simulink model "example_3DOF_2"  (R2019a)
settings: Solver=ode45  StartTime=0.0  StopTime=250  RelTol=1e-5
PostLoadFcn:
  | flightControlCallback('initializeParameters', bdroot, '3DOF', 0);
InitFcn:
  | flightControlCallback('runSim', bdroot);
undefined symbols (not defined in the file or in its folder): aeroCoeff, vehicle
libraries: aerolibasang x3, shared3dof x1, sharedtransform x1
settings Model: Creator=Devansh  LastModifiedBy=Devansh
settings SolverCC: MinimalZcImpactIntegration=on
settings DataIOCC: ExternalInput=getinputstruct(op);  InitialState=getstatestruct(op);  SaveFormat=Array
settings OptimizationCC: EnhancedBackFolding=on  StrengthReduction=on  InitFltsAndDblsToZero=on  DifferentSizesBufferReuse=on
settings DebuggingCC: WriteAfterWriteMsg=DisableAll  AlgebraicLoopMsg=none  FcnCallInpInsideContextMsg=warning  UnconnectedInputMsg=none  UnconnectedOutputMsg=none  UnconnectedLineMsg=none  UniqueDataStoreMsg=error  StateNameClashWarn=warning  PregeneratedLibrarySubsystemCodeDiagnostic=none  StrictBusMsg=ErrorOnBusTreatedAsVector  SFUnexpectedBacktrackingDiag=warning  SFNoUnconditionalDefaultTransitionDiag=warning  SFExecutionAtInitializationDiag=none  ArithmeticOperatorsInVariantConditions=warning
settings ModelReferenceCC: PropagateSignalLabelsOutOfModel=off
settings SFSimCC: SimUseLocalCustomCode=off
settings RTWCC: RTWUseLocalCustomCode=off
settings CodeAppCC: StateflowObjectComments=on

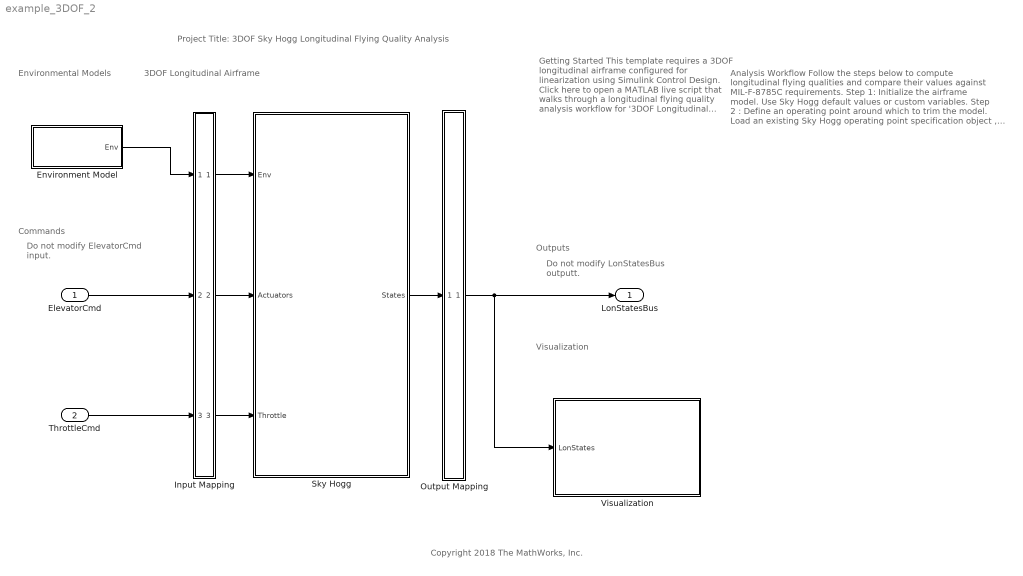
== system example_3DOF_2 ==
  note: Do not modify ElevatorCmd input.
  note: Project Title: 3DOF Sky Hogg Longitudinal Flying Quality Analysis
  note: Analysis Workflow
      | Follow the steps below to compute longitudinal flying qualities and compare their values against MIL-F-8785C requirements.
      |
      | Step 1: Initialize the airframe model. Use Sky Hogg default values or custom variables.
      |
      | Step 2 : Define an operating point around which to trim the model. Load an existing Sky Hogg operating point specification object , or launch the Linear Analysis Trim Tool to create a new one . You must use the 'Export' button in the dialog window to save your opCond.OperatingSpec object to the base workspace.
      |
      | Step 3: Trim the airframe model around a given operating point specification. (Optional:) Initialize the model with the trim inputs and states. Simulate the model to confirm steady-state behavior, then undo initialization.
      |
      | Step 4: Linearize the airframe dynamics around a trimmed operating point using the linear analysis input and output points defined in the model. You can modify linear analysis points by right-clicking on a signal line, and navigating to "Linear Analysis Points".
      |
      | Step 5: Compute longitudinal handling qualities (phugoid mode and short-period mode characteristics) for a linear airframe model using eigenvalue analysis, and compare the results against MIL-F-8785C requirements.
  note: Copyright 2018 The MathWorks, Inc.
  note: 3DOF Longitudinal Airframe
  note: Environmental Models
  note: Commands
  note: Visualization
  note: Outputs
  note: Getting Started
      | This template requires a 3DOF longitudinal airframe configured for linearization using Simulink Control Design.
      |
      | Click here to open a MATLAB live script that walks through a longitudinal flying quality analysis workflow for '3DOF Longitudinal Airframe' Simulink template .
  note: Do not modify LonStatesBus outputt.
  ElevatorCmd : Inport  OutDataTypeStr=double
  ThrottleCmd : Inport  Port=2  OutDataTypeStr=double
  Environment Model : Subsystem
  Input Mapping : Subsystem
  Output Mapping : Subsystem
  Sky Hogg : Subsystem
      settings: AttributesFormatString=|
      | Must contain one 3DOF
      | (Body Axis) block
  Visualization : Subsystem
  LonStatesBus : Outport
  wires:
  Sky Hogg/1(States) -> Output Mapping/1(StatesIn)
  Environment Model/1(Env) -> Input Mapping/1(EnvironmentIn)
  ElevatorCmd/1 -> Input Mapping/2(ActuatorCmds)
  ThrottleCmd/1 -> Input Mapping/3(ThrottleIn)
  Input Mapping/3(ThrottleOut) -> Sky Hogg/3(Throttle)
  Input Mapping/2(ActuatorCmdsOut) -> Sky Hogg/2(Actuators)
  Input Mapping/1(EnvironmentOut) -> Sky Hogg/1(Env)
  Output Mapping/1(StatesOut) -> Visualization/1(LonStates), LonStatesBus/1

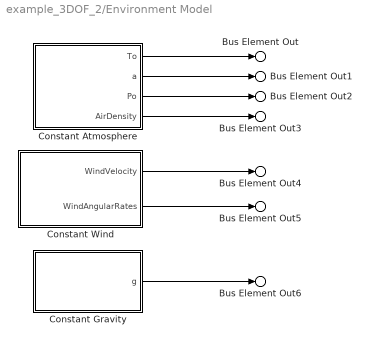
== system example_3DOF_2/Environment Model ==
  Constant Atmosphere : Subsystem  VariantControl=atmosCONST  mask(Standard Atmospheric Constants){To=275.15, a=332.529, Po=79495.2, AirDensity=1.00649}
      mask prompts: To "Constant Temperature (K):"; a "Constant Speed of Sound (m/s):"; Po "Constant Pressure (Pa):"; AirDensity "Constant Air Density (kg/m^3):"
  Constant Gravity : Subsystem  VariantControl=gravCONST  mask(Constant Gravitational Acceleration){g=[0 0 9.80665]}
      mask prompts: g "Constant Gravitational Acceleration (m/s^2):"
  Constant Wind : Subsystem  VariantControl=windCONST  mask(Constant Wind Values){ugvgwg=[-2 0 -1], pgqgrg=[0 0 0]}
      mask prompts: ugvgwg "Constant Wind Velocity (m/s):"; pgqgrg "Constant Wind Angular Rates (rad/s):"
  Bus Element Out : Outport  PortName=Env  Element=To
  Bus Element Out1 : Outport  PortName=Env  Element=a
  Bus Element Out2 : Outport  PortName=Env  Element=Po
  Bus Element Out3 : Outport  PortName=Env  Element=AirDensity
  Bus Element Out4 : Outport  PortName=Env  Element=WindVelocity
  Bus Element Out5 : Outport  PortName=Env  Element=WindAngularRates
  Bus Element Out6 : Outport  PortName=Env  Element=g
  wires:
  Constant Gravity/1(g) -> Bus Element Out6/1
  Constant Atmosphere/2(a) -> Bus Element Out1/1
  Constant Wind/1(WindVelocity) -> Bus Element Out4/1
  Constant Atmosphere/1(To) -> Bus Element Out/1
  Constant Atmosphere/4(AirDensity) -> Bus Element Out3/1
  Constant Atmosphere/3(Po) -> Bus Element Out2/1
  Constant Wind/2(WindAngularRates) -> Bus Element Out5/1

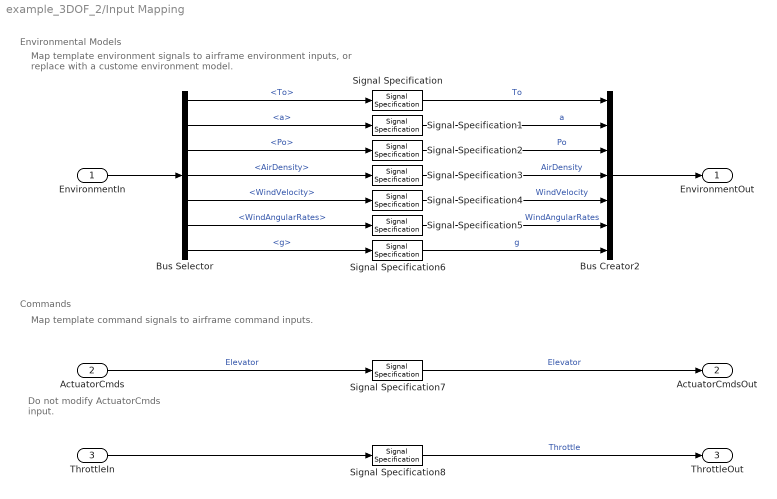
== system example_3DOF_2/Input Mapping ==
  note: Map template environment signals to airframe environment inputs, or replace with a custome environment model.
  note: Map template command signals to airframe command inputs.
  note: Commands
  note: Environmental Models
  note: Do not modify ActuatorCmds input.
  EnvironmentIn : Inport
  ActuatorCmds : Inport  Port=2
  ThrottleIn : Inport  Port=3
  Bus Creator2 : BusCreator  Inputs=7
  Bus Selector : BusSelector  OutputSignals=To,a,Po,AirDensity,WindVelocity,WindAngularRates,g
  Signal Specification{,1..8} (9 alike) : SignalSpecification  OutDataTypeStr=double
  EnvironmentOut : Outport
  ActuatorCmdsOut : Outport  Port=2
  ThrottleOut : Outport  Port=3
  wires:
  EnvironmentIn/1 -> Bus Selector/1
  Bus Creator2/1 -> EnvironmentOut/1
  ThrottleIn/1 -> Signal Specification8/1
  Bus Selector/1 -> Signal Specification/1  "<To>"
  Bus Selector/2 -> Signal Specification1/1  "<a>"
  Bus Selector/3 -> Signal Specification2/1  "<Po>"
  Bus Selector/4 -> Signal Specification3/1  "<AirDensity>"
  Bus Selector/5 -> Signal Specification4/1  "<WindVelocity>"
  Bus Selector/6 -> Signal Specification5/1  "<WindAngularRates>"
  Bus Selector/7 -> Signal Specification6/1  "<g>"
  ActuatorCmds/1 -> Signal Specification7/1  "Elevator"
  Signal Specification2/1 -> Bus Creator2/3  "Po"
  Signal Specification3/1 -> Bus Creator2/4  "AirDensity"
  Signal Specification6/1 -> Bus Creator2/7  "g"
  Signal Specification4/1 -> Bus Creator2/5  "WindVelocity"
  Signal Specification5/1 -> Bus Creator2/6  "WindAngularRates"
  Signal Specification/1 -> Bus Creator2/1  "To"
  Signal Specification1/1 -> Bus Creator2/2  "a"
  Signal Specification7/1 -> ActuatorCmdsOut/1  "Elevator"
  Signal Specification8/1 -> ThrottleOut/1  "Throttle"

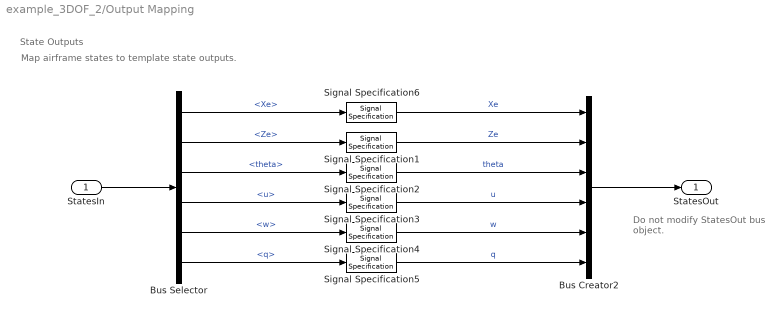
== system example_3DOF_2/Output Mapping ==
  note: State Outputs
  note: Map airframe states to template state outputs.
  note: Do not modify StatesOut bus object.
  StatesIn : Inport
  Bus Creator2 : BusCreator  Inputs=6
  Bus Selector : BusSelector  OutputSignals=Xe,Ze,theta,u,w,q
  Signal Specification{1..6} (6 alike) : SignalSpecification  OutDataTypeStr=double
  StatesOut : Outport  OutDataTypeStr=Bus: flightControl3DOFStatesBus
  wires:
  Bus Creator2/1 -> StatesOut/1
  StatesIn/1 -> Bus Selector/1
  Bus Selector/1 -> Signal Specification6/1  "<Xe>"
  Bus Selector/2 -> Signal Specification1/1  "<Ze>"
  Bus Selector/3 -> Signal Specification2/1  "<theta>"
  Bus Selector/4 -> Signal Specification3/1  "<u>"
  Bus Selector/5 -> Signal Specification4/1  "<w>"
  Bus Selector/6 -> Signal Specification5/1  "<q>"
  Signal Specification6/1 -> Bus Creator2/1  "Xe"
  Signal Specification1/1 -> Bus Creator2/2  "Ze"
  Signal Specification2/1 -> Bus Creator2/3  "theta"
  Signal Specification3/1 -> Bus Creator2/4  "u"
  Signal Specification4/1 -> Bus Creator2/5  "w"
  Signal Specification5/1 -> Bus Creator2/6  "q"

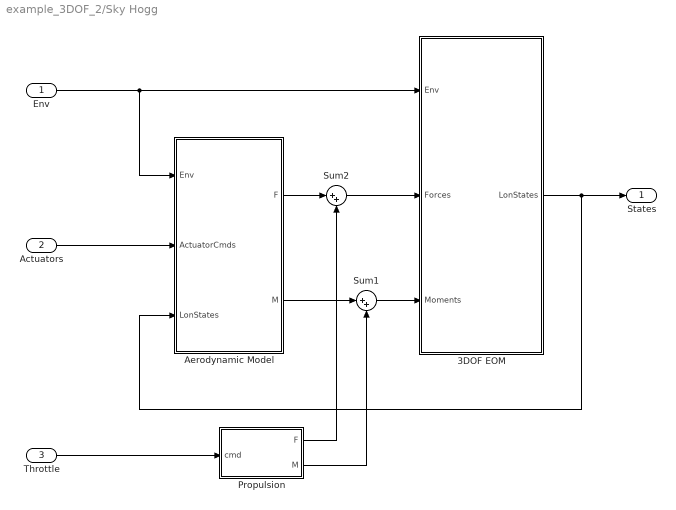
== system example_3DOF_2/Sky Hogg ==
  Env : Inport
  Actuators : Inport  Port=2
  Throttle : Inport  Port=3
  3DOF EOM : Subsystem  VariantControl=eom3DOF
      settings: AttributesFormatString=|
      | Must contain one 3DOF
      | (Body Axis) block
  Aerodynamic Model : Subsystem  VariantControl=aeroCONST
  Propulsion : Subsystem
      settings: RTWSystemCode=Inline
  Sum1 : Sum  Inputs=|++  SaturateOnIntegerOverflow=on  InputSameDT=on  OutDataTypeStr=Inherit: Same as first input
  Sum2 : Sum  Inputs=|++  SaturateOnIntegerOverflow=on  InputSameDT=on  OutDataTypeStr=Inherit: Same as first input
  States : Outport
  wires:
  Actuators/1 -> Aerodynamic Model/2(ActuatorCmds)
  Aerodynamic Model/1(F) -> Sum2/1
  Propulsion/1(F) -> Sum2/2
  Sum1/1 -> 3DOF EOM/3(Moments)
  Env/1 -> Aerodynamic Model/1(Env), 3DOF EOM/1(Env)
  Propulsion/2(M) -> Sum1/2
  Aerodynamic Model/2(" M") -> Sum1/1
  Sum2/1 -> 3DOF EOM/2(Forces)
  3DOF EOM/1(LonStates) -> Aerodynamic Model/3(LonStates), States/1
  Throttle/1 -> Propulsion/1(cmd)

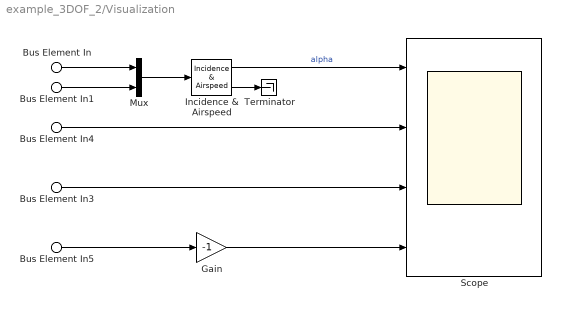
== system example_3DOF_2/Visualization ==
  Bus Element In : Inport  PortName=LonStates  Element=u
  Bus Element In1 : Inport  PortName=LonStates  Element=w
  Bus Element In3 : Inport  PortName=LonStates  Element=q
  Bus Element In4 : Inport  PortName=LonStates  Element=theta
  Bus Element In5 : Inport  PortName=LonStates  Element=Ze
  Gain : Gain  Gain=-1
  Incidence & Airspeed : aerolibasang/Incidence  & Airspeed
      settings: SourceProductName=Aerospace Blockset  SourceProductBaseCode=AE
  Mux : Mux  Inputs=2
  Scope : Scope  NumInputPorts=4
  Terminator : Terminator
  wires:
  Incidence & Airspeed/1 -> Scope/1  "alpha"
  Incidence & Airspeed/2 -> Terminator/1
  Bus Element In/1 -> Mux/1
  Bus Element In1/1 -> Mux/2
  Mux/1 -> Incidence & Airspeed/1
  Bus Element In3/1 -> Scope/3
  Bus Element In4/1 -> Scope/2
  Bus Element In5/1 -> Gain/1
  Gain/1 -> Scope/4

== system example_3DOF_2/Environment Model/Constant Atmosphere ==
  Constant : Constant  Value=To
  Constant1 : Constant  Value=a
  Constant2 : Constant  Value=Po
  Constant3 : Constant  Value=AirDensity
  To : Outport
  a : Outport  Port=2
  Po : Outport  Port=3
  AirDensity : Outport  Port=4
  wires:
  Constant3/1 -> AirDensity/1
  Constant2/1 -> Po/1
  Constant/1 -> To/1
  Constant1/1 -> a/1

== system example_3DOF_2/Environment Model/Constant Gravity ==
  Reshape1 : Reshape  OutputDimensionality=Column vector (2-D)
  Standard Gravity : Constant  Value=g
  g : Outport
  wires:
  Standard Gravity/1 -> Reshape1/1
  Reshape1/1 -> g/1

== system example_3DOF_2/Environment Model/Constant Wind ==
  Reshape : Reshape  OutputDimensionality=Column vector (2-D)
  Reshape1 : Reshape  OutputDimensionality=Column vector (2-D)
  pg,qg,rg : Constant  Value=pgqgrg
  ug,vg,wg : Constant  Value=ugvgwg
  WindVelocity : Outport
  WindAngularRates : Outport  Port=2
  wires:
  Reshape1/1 -> WindAngularRates/1
  Reshape/1 -> WindVelocity/1
  ug,vg,wg/1 -> Reshape/1
  pg,qg,rg/1 -> Reshape1/1

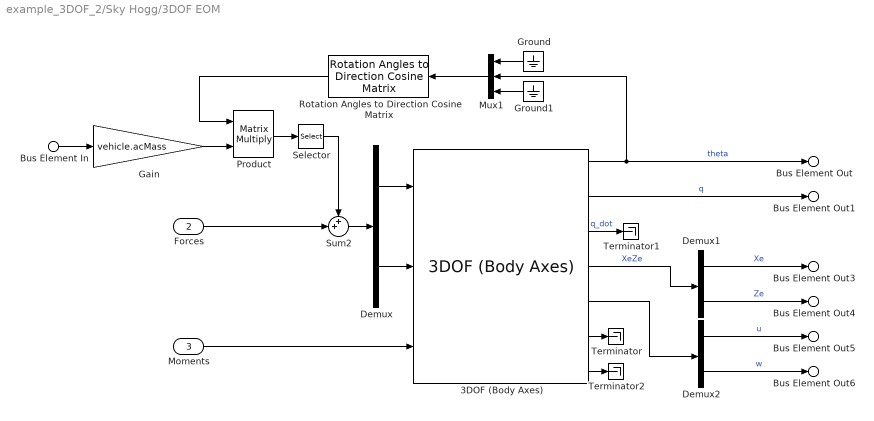
== system example_3DOF_2/Sky Hogg/3DOF EOM ==
  Bus Element In : Inport  PortName=Env  Element=g
  Forces : Inport  Port=2
  Moments : Inport  Port=3
  3DOF (Body Axes) : shared3dof/3DOF (Body Axes)  units=Metric (MKS)  mtype=Fixed  v_ini=initCond.v0  theta_ini=initCond.theta0  alpha_ini=initCond.alpha0  pos_ini=initCond.x0  q_ini=initCond.q0  mass=vehicle.acMass  mass_e=0.5  mass_f=3.0  Iyy=vehicle.inertia_yy  Iyy_e=0.5  Iyy_f=3.0  g_in=Internal  g=0  vre_flag=on  abi_flag=on  aMode=0  vel_statename={'u', 'w'}  theta_statename='theta'  pos_statename={'Xe', 'Ze'}  q_statename='q'  mass_statename=''
      settings: SourceProductName=Aerospace Blockset  SourceProductBaseCode=AE
  Demux : Demux  Outputs=2
  Demux1 : Demux  Outputs=2
  Demux2 : Demux  Outputs=2
  Gain : Gain  Gain=vehicle.acMass
  Ground : Ground
  Ground1 : Ground
  Mux1 : Mux  Inputs=3
  Product : Product  Multiplication=Matrix(*)
  Rotation Angles to Direction Cosine Matrix : sharedtransform/Rotation Angles to Direction Cosine Matrix  rotationOrder=ZYX  aMode=aMode
      settings: SourceProductBaseCode=AE
  Selector : Selector  InputPortWidth=3  IndexOptions=Index vector (dialog)  Indices=[1 3]  OutputSizes=1
  Sum2 : Sum  Inputs=++|  SaturateOnIntegerOverflow=on  InputSameDT=on  OutDataTypeStr=Inherit: Same as first input
  Terminator : Terminator
  Terminator1 : Terminator
  Terminator2 : Terminator
  Bus Element Out : Outport  PortName=LonStates  Element=theta
  Bus Element Out1 : Outport  PortName=LonStates  Element=q
  Bus Element Out3 : Outport  PortName=LonStates  Element=Xe
  Bus Element Out4 : Outport  PortName=LonStates  Element=Ze
  Bus Element Out5 : Outport  PortName=LonStates  Element=u
  Bus Element Out6 : Outport  PortName=LonStates  Element=w
  wires:
  3DOF (Body Axes)/6 -> Terminator/1
  Demux1/1 -> Bus Element Out3/1  "Xe"
  Demux1/2 -> Bus Element Out4/1  "Ze"
  Demux2/1 -> Bus Element Out5/1  "u"
  Demux2/2 -> Bus Element Out6/1  "w"
  3DOF (Body Axes)/5 -> Demux2/1
  3DOF (Body Axes)/4 -> Demux1/1  "XeZe"
  3DOF (Body Axes)/2 -> Bus Element Out1/1  "q"
  3DOF (Body Axes)/1 -> Bus Element Out/1, Mux1/2  "theta"
  Moments/1 -> 3DOF (Body Axes)/3
  Bus Element In/1 -> Gain/1
  Forces/1 -> Sum2/2
  Product/1 -> Selector/1
  Rotation Angles to Direction Cosine Matrix/1 -> Product/1
  Gain/1 -> Product/2
  Mux1/1 -> Rotation Angles to Direction Cosine Matrix/1
  Ground/1 -> Mux1/1
  Ground1/1 -> Mux1/3
  Selector/1 -> Sum2/1
  Sum2/1 -> Demux/1
  Demux/1 -> 3DOF (Body Axes)/1
  Demux/2 -> 3DOF (Body Axes)/2
  3DOF (Body Axes)/3 -> Terminator1/1  "q_dot"
  3DOF (Body Axes)/7 -> Terminator2/1

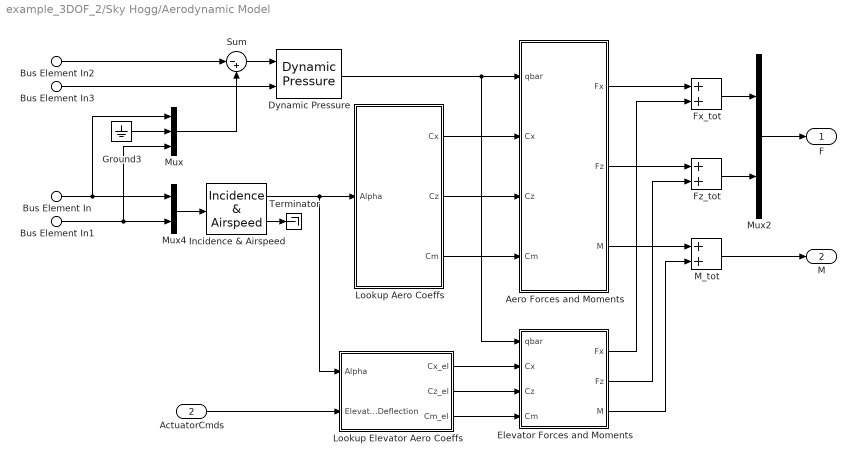
== system example_3DOF_2/Sky Hogg/Aerodynamic Model ==
  Bus Element In2 : Inport  PortName=Env  Element=WindVelocity
  Bus Element In3 : Inport  PortName=Env  Element=AirDensity
  ActuatorCmds : Inport  Port=2
  Bus Element In : Inport  Port=3  PortName=LonStates  Element=u
  Bus Element In1 : Inport  Port=3  PortName=LonStates  Element=w
  Aero Forces and Moments : Subsystem
  Dynamic Pressure : aerolibasang/Dynamic Pressure
  Elevator Forces and Moments : Subsystem
  Fx_tot : Sum  SaturateOnIntegerOverflow=on  InputSameDT=on  OutDataTypeStr=Inherit: Same as first input
  Fz_tot : Sum  SaturateOnIntegerOverflow=on  InputSameDT=on  OutDataTypeStr=Inherit: Same as first input
  Ground3 : Ground
  Incidence & Airspeed : aerolibasang/Incidence  & Airspeed
      settings: SourceProductName=Aerospace Blockset  SourceProductBaseCode=AE
  Lookup Aero Coeffs : Subsystem
  Lookup Elevator Aero Coeffs : Subsystem
  M_tot : Sum  SaturateOnIntegerOverflow=on  InputSameDT=on  OutDataTypeStr=Inherit: Same as first input
  Mux : Mux  Inputs=3
  Mux2 : Mux  Inputs=2
  Mux4 : Mux  Inputs=2
  Sum : Sum  Inputs=|-+
  Terminator : Terminator
  F : Outport
  " M" : Outport  Port=2  Unit=N*m
  wires:
  Fz_tot/1 -> Mux2/2
  Fx_tot/1 -> Mux2/1
  Aero Forces and Moments/2(Fz) -> Fz_tot/1
  Elevator Forces and Moments/2(Fz) -> Fz_tot/2
  Elevator Forces and Moments/1(Fx) -> Fx_tot/2
  Lookup Elevator Aero Coeffs/3(Cm_el) -> Elevator Forces and Moments/4(Cm)
  Lookup Elevator Aero Coeffs/2(Cz_el) -> Elevator Forces and Moments/3(Cz)
  Lookup Elevator Aero Coeffs/1(Cx_el) -> Elevator Forces and Moments/2(Cx)
  Lookup Aero Coeffs/3(Cm) -> Aero Forces and Moments/4(Cm)
  Lookup Aero Coeffs/2(Cz) -> Aero Forces and Moments/3(Cz)
  Lookup Aero Coeffs/1(Cx) -> Aero Forces and Moments/2(Cx)
  Aero Forces and Moments/3(M) -> M_tot/1
  Aero Forces and Moments/1(Fx) -> Fx_tot/1
  Dynamic Pressure/1 -> Aero Forces and Moments/1(qbar), Elevator Forces and Moments/1(qbar)
  Elevator Forces and Moments/3(M) -> M_tot/2
  Mux/1 -> Sum/2
  Incidence & Airspeed/1 -> Lookup Elevator Aero Coeffs/1(Alpha), Lookup Aero Coeffs/1(Alpha)
  Sum/1 -> Dynamic Pressure/1
  ActuatorCmds/1 -> Lookup Elevator Aero Coeffs/2(Elevator Deflection)
  M_tot/1 -> " M"/1
  Ground3/1 -> Mux/2
  Mux4/1 -> Incidence & Airspeed/1
  Mux2/1 -> F/1
  Bus Element In1/1 -> Mux/3, Mux4/2
  Bus Element In/1 -> Mux/1, Mux4/1
  Incidence & Airspeed/2 -> Terminator/1
  Bus Element In2/1 -> Sum/1
  Bus Element In3/1 -> Dynamic Pressure/2

== system example_3DOF_2/Sky Hogg/Propulsion ==
  cmd : Inport
  Mux : Mux  Inputs=2
  ThrustX : Lookup_n-D  NumberOfTableDimensions=1  LookupTableObject=''  BreakpointsForDimension1=(1/6)*(3+([-3:3]))  IndexSearchMethod=Linear search  BeginIndexSearchUsingPreviousIndexResult=on  Table=vehicle.Thrust*(1+tanh([-3:3]))  ExtrapMethod=Clip  InputSameDT=on
  ThrustZ : Constant  Value=0  SampleTime=-1
  Thrust_M : Constant  Value=0  SampleTime=-1
  F : Outport  Unit=N
  M : Outport  Port=2  Unit=N*m
  wires:
  ThrustX/1 -> Mux/1
  ThrustZ/1 -> Mux/2
  Mux/1 -> F/1
  Thrust_M/1 -> M/1
  cmd/1 -> ThrustX/1

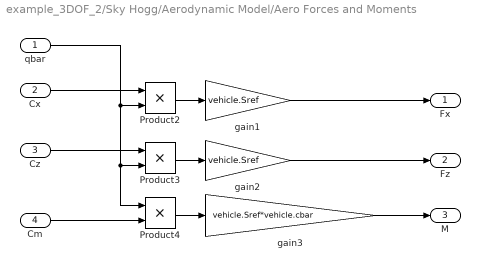
== system example_3DOF_2/Sky Hogg/Aerodynamic Model/Aero Forces and Moments ==
  qbar : Inport
  Cx : Inport  Port=2
  Cz : Inport  Port=3
  Cm : Inport  Port=4
  Product2 : Product  SaturateOnIntegerOverflow=on  InputSameDT=on  OutDataTypeStr=Inherit: Same as first input
  Product3 : Product  SaturateOnIntegerOverflow=on  InputSameDT=on  OutDataTypeStr=Inherit: Same as first input
  Product4 : Product  SaturateOnIntegerOverflow=on  InputSameDT=on  OutDataTypeStr=Inherit: Same as first input
  gain1 : Gain  Gain=vehicle.Sref  SaturateOnIntegerOverflow=on  OutDataTypeStr=Inherit: Same as input  ParamDataTypeStr=Inherit: Same as input
  "gain2 " : Gain  Gain=vehicle.Sref  SaturateOnIntegerOverflow=on  OutDataTypeStr=Inherit: Same as input  ParamDataTypeStr=Inherit: Same as input
  gain3 : Gain  Gain=vehicle.Sref*vehicle.cbar  SaturateOnIntegerOverflow=on  OutDataTypeStr=Inherit: Same as input  ParamDataTypeStr=Inherit: Same as input
  Fx : Outport
  Fz : Outport  Port=2
  M : Outport  Port=3
  wires:
  gain1/1 -> Fx/1
  Cx/1 -> Product2/1
  Cz/1 -> Product3/1
  Product3/1 -> "gain2 "/1
  Cm/1 -> Product4/2
  Product2/1 -> gain1/1
  Product4/1 -> gain3/1
  qbar/1 -> Product3/2, Product4/1, Product2/2
  "gain2 "/1 -> Fz/1
  gain3/1 -> M/1

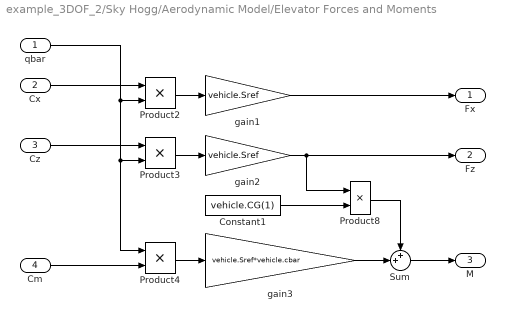
== system example_3DOF_2/Sky Hogg/Aerodynamic Model/Elevator Forces and Moments ==
  qbar : Inport
  Cx : Inport  Port=2
  Cz : Inport  Port=3
  Cm : Inport  Port=4
  Constant1 : Constant  Value=vehicle.CG(1)
  Product2 : Product  SaturateOnIntegerOverflow=on  InputSameDT=on  OutDataTypeStr=Inherit: Same as first input
  Product3 : Product  SaturateOnIntegerOverflow=on  InputSameDT=on  OutDataTypeStr=Inherit: Same as first input
  Product4 : Product  SaturateOnIntegerOverflow=on  InputSameDT=on  OutDataTypeStr=Inherit: Same as first input
  Product8 : Product
  Sum : Sum  Inputs=++|
  gain1 : Gain  Gain=vehicle.Sref  SaturateOnIntegerOverflow=on  OutDataTypeStr=Inherit: Same as input  ParamDataTypeStr=Inherit: Same as input
  "gain2 " : Gain  Gain=vehicle.Sref  SaturateOnIntegerOverflow=on  OutDataTypeStr=Inherit: Same as input  ParamDataTypeStr=Inherit: Same as input
  gain3 : Gain  Gain=vehicle.Sref*vehicle.cbar  SaturateOnIntegerOverflow=on  OutDataTypeStr=Inherit: Same as input  ParamDataTypeStr=Inherit: Same as input
  Fx : Outport
  Fz : Outport  Port=2
  M : Outport  Port=3
  wires:
  qbar/1 -> Product4/1, Product3/2, Product2/2
  Product4/1 -> gain3/1
  Product2/1 -> gain1/1
  Cm/1 -> Product4/2
  Product3/1 -> "gain2 "/1
  Cz/1 -> Product3/1
  Cx/1 -> Product2/1
  gain1/1 -> Fx/1
  gain3/1 -> Sum/2
  Product8/1 -> Sum/1
  Constant1/1 -> Product8/2
  "gain2 "/1 -> Fz/1, Product8/1
  Sum/1 -> M/1

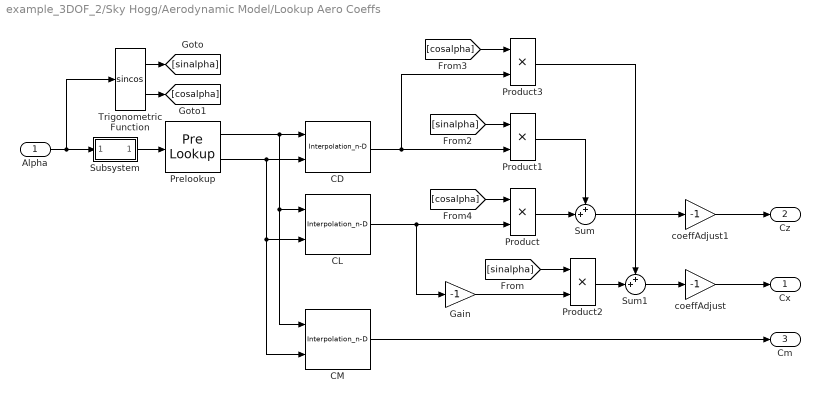
== system example_3DOF_2/Sky Hogg/Aerodynamic Model/Lookup Aero Coeffs ==
  Alpha : Inport  Unit=rad
  CD : Interpolation_n-D  NumberOfTableDimensions=1  Table=aeroCoeff.CD  InternalRulePriority=Speed
      settings: InputPortMap=u0,u1
  CL : Interpolation_n-D  NumberOfTableDimensions=1  Table=aeroCoeff.CL  InternalRulePriority=Speed
      settings: InputPortMap=u0,u1
  CM : Interpolation_n-D  NumberOfTableDimensions=1  Table=aeroCoeff.CM  InternalRulePriority=Speed
      settings: InputPortMap=u0,u1
  Gain : Gain  Gain=-1
  Prelookup : PreLookup  BreakpointsData=aeroCoeff.alpha_vec  ExtrapMethod=Linear
  Product{,1..3} (4 alike) : Product
  Subsystem : Subsystem
      mask Display:
      | port_label('output',1,'deg')
      | port_label('input',1,'rad')
  Sum : Sum  Inputs=++|
  Sum1 : Sum  Inputs=++|
  Trigonometric Function : Trigonometry  Operator=sincos
  coeffAdjust : Gain  Gain=-1
  coeffAdjust1 : Gain  Gain=-1
  Cx : Outport
  Cz : Outport  Port=2
  Cm : Outport  Port=3
  wires:
  CL/1 -> Gain/1, Product/2
  CM/1 -> Cm/1
  Prelookup/1 -> CM/1, CL/1, CD/1
  Prelookup/2 -> CM/2, CL/2, CD/2
  Product/1 -> Sum/2
  CD/1 -> Product3/2, Product1/2
  Product1/1 -> Sum/1
  Sum/1 -> coeffAdjust1/1
  Gain/1 -> Product2/2
  Product2/1 -> Sum1/2
  Product3/1 -> Sum1/1
  Sum1/1 -> coeffAdjust/1
  coeffAdjust1/1 -> Cz/1
  coeffAdjust/1 -> Cx/1
  Alpha/1 -> Trigonometric Function/1, Subsystem/1(In1)
  [sinalpha] -> Product2/1
  [sinalpha] -> Product1/1
  [cosalpha] -> Product3/1
  [cosalpha] -> Product/1
  Trigonometric Function/2 -> [cosalpha]
  Trigonometric Function/1 -> [sinalpha]
  Subsystem/1(Out2) -> Prelookup/1

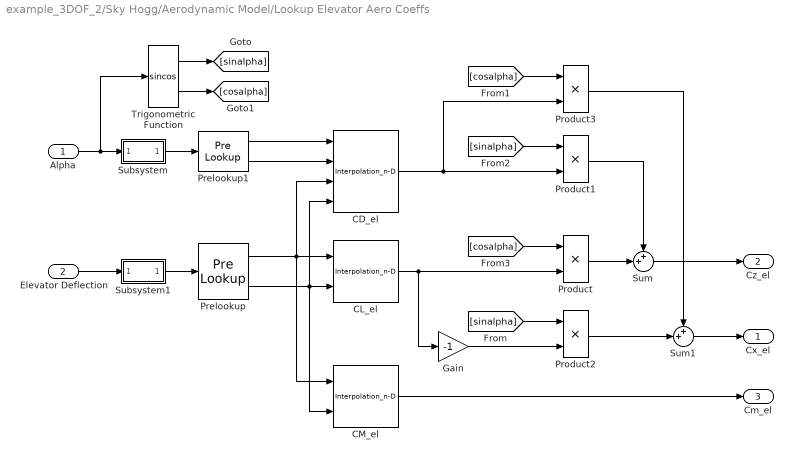
== system example_3DOF_2/Sky Hogg/Aerodynamic Model/Lookup Elevator Aero Coeffs ==
  Alpha : Inport  Unit=rad
  Elevator Deflection : Inport  Port=2  Unit=rad
  CD_el : Interpolation_n-D  Table=aeroCoeff.CD_el
  CL_el : Interpolation_n-D  NumberOfTableDimensions=1  Table=aeroCoeff.CL_el  InternalRulePriority=Speed
      settings: InputPortMap=u0,u1
  CM_el : Interpolation_n-D  NumberOfTableDimensions=1  Table=aeroCoeff.CM_el  InternalRulePriority=Speed
      settings: InputPortMap=u0,u1
  Gain : Gain  Gain=-1
  Prelookup : PreLookup  BreakpointsData=aeroCoeff.def_vec  ExtrapMethod=Linear  IndexDataTypeStr=int32  FractionDataTypeStr=double
  Prelookup1 : PreLookup  BreakpointsData=aeroCoeff.alpha_vec  ExtrapMethod=Linear  IndexDataTypeStr=int32  FractionDataTypeStr=double
  Product{,1..3} (4 alike) : Product
  Subsystem : Subsystem
      mask Display:
      | port_label('output',1,'deg')
      | port_label('input',1,'rad')
  Subsystem1 : Subsystem
      mask Display:
      | port_label('output',1,'deg')
      | port_label('input',1,'rad')
  Sum : Sum  Inputs=++|
  Sum1 : Sum  Inputs=++|
  Trigonometric Function : Trigonometry  Operator=sincos
  Cx_el : Outport
  Cz_el : Outport  Port=2
  Cm_el : Outport  Port=3
  wires:
  Sum1/1 -> Cx_el/1
  CM_el/1 -> Cm_el/1
  Sum/1 -> Cz_el/1
  Product1/1 -> Sum/1
  Product/1 -> Sum/2
  Product2/1 -> Sum1/2
  CL_el/1 -> Product/2, Gain/1
  Product3/1 -> Sum1/1
  Gain/1 -> Product2/2
  CD_el/1 -> Product1/2, Product3/2
  Prelookup/1 -> CM_el/1, CL_el/1, CD_el/3
  Prelookup/2 -> CD_el/4, CL_el/2, CM_el/2
  Alpha/1 -> Subsystem/1(In1), Trigonometric Function/1
  Subsystem/1(Out2) -> Prelookup1/1
  Elevator Deflection/1 -> Subsystem1/1(In1)
  Prelookup1/1 -> CD_el/1
  Prelookup1/2 -> CD_el/2
  [sinalpha] -> Product2/1
  [sinalpha] -> Product1/1
  [cosalpha] -> Product3/1
  [cosalpha] -> Product/1
  Trigonometric Function/2 -> [cosalpha]
  Trigonometric Function/1 -> [sinalpha]
  Subsystem1/1(Out2) -> Prelookup/1

== system example_3DOF_2/Sky Hogg/Aerodynamic Model/Lookup Aero Coeffs/Subsystem ==
  In1 : Inport
  Signal Specification : SignalSpecification  Unit=deg
  Unit Conversion : UnitConversion
  Out2 : Outport
  wires:
  Signal Specification/1 -> Out2/1
  Unit Conversion/1 -> Signal Specification/1
  In1/1 -> Unit Conversion/1

== system example_3DOF_2/Sky Hogg/Aerodynamic Model/Lookup Elevator Aero Coeffs/Subsystem ==
  In1 : Inport
  Signal Specification : SignalSpecification  Unit=deg
  Unit Conversion : UnitConversion
  Out2 : Outport
  wires:
  Signal Specification/1 -> Out2/1
  Unit Conversion/1 -> Signal Specification/1
  In1/1 -> Unit Conversion/1

== system example_3DOF_2/Sky Hogg/Aerodynamic Model/Lookup Elevator Aero Coeffs/Subsystem1 ==
  In1 : Inport
  Signal Specification : SignalSpecification  Unit=deg
  Unit Conversion : UnitConversion
  Out2 : Outport
  wires:
  In1/1 -> Unit Conversion/1
  Unit Conversion/1 -> Signal Specification/1
  Signal Specification/1 -> Out2/1
